simulink model "Test_MotionSM"  (R2017b)
settings: Solver=FixedStepAuto  StartTime=0.0  StopTime=inf  FixedStep=0.00001  RelTol=1e-3
model workspace (MAT data in the model file):
  AP = Simulink.Signal
  AP.DataType = 'double'
  AP.Dimensions = 1
  AP.DimensionsMode = 'Fixed'
  AP.Complexity = 'real'
  AP.SampleTime = -1
  AP.SamplingMode = 'auto'
  ZZP = Simulink.Signal
  ZZP.DataType = 'double'
  ZZP.Dimensions = 1
  ZZP.DimensionsMode = 'Fixed'
  ZZP.Complexity = 'real'
  ZZP.SampleTime = -1
  ZZP.SamplingMode = 'auto'
  ZZP.InitialValue = '0'
  ZZP_wait = Simulink.Signal
  ZZP_wait.DataType = 'double'
  ZZP_wait.Dimensions = 1
  ZZP_wait.DimensionsMode = 'Fixed'
  ZZP_wait.Complexity = 'real'
  ZZP_wait.SampleTime = -1
  ZZP_wait.SamplingMode = 'auto'
  ZZP_wait.InitialValue = '0'
settings Model: Creator=张紫薇  LastModifiedBy=张紫薇

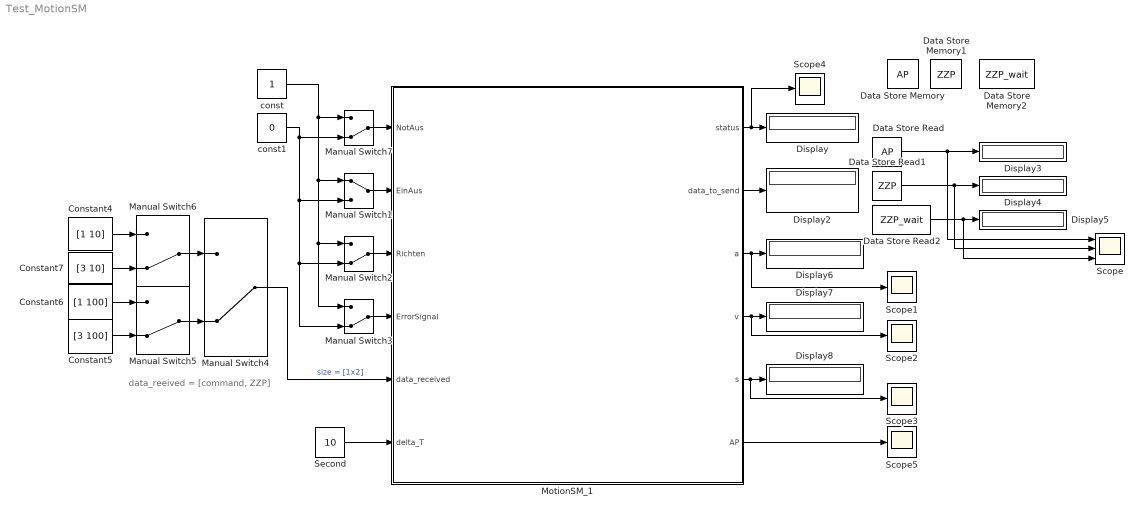
== system Test_MotionSM ==
  note: data_reeived = [command, ZZP]
  Constant4 : Constant  Value=[1 10]  OutDataTypeStr=double
  Constant5 : Constant  Value=[3 100]  OutDataTypeStr=double
  Constant6 : Constant  Value=[1 100]  OutDataTypeStr=double
  Constant7 : Constant  Value=[3 10]  OutDataTypeStr=double
  Data Store Memory : DataStoreMemory  DataStoreName=AP  ReadBeforeWriteMsg=warning  WriteAfterWriteMsg=warning  WriteAfterReadMsg=warning  ShowAdditionalParam=off  OutMin=[0]  OutMax=[100]  OutDataTypeStr=double  Dimensions=1
  Data Store Memory1 : DataStoreMemory  DataStoreName=ZZP  ReadBeforeWriteMsg=warning  WriteAfterWriteMsg=warning  WriteAfterReadMsg=warning  ShowAdditionalParam=off  OutDataTypeStr=double  Dimensions=1
  Data Store Memory2 : DataStoreMemory  DataStoreName=ZZP_wait  ReadBeforeWriteMsg=warning  WriteAfterWriteMsg=warning  WriteAfterReadMsg=warning  ShowAdditionalParam=off  OutDataTypeStr=double  Dimensions=1
  Data Store Read : DataStoreRead  DataStoreName=AP
  Data Store Read1 : DataStoreRead  DataStoreName=ZZP
  Data Store Read2 : DataStoreRead  DataStoreName=ZZP_wait
  Display{,2..8} (8 alike) : Display
      Display3 settings: Format=decimal (Stored Integer)
      Display4 settings: Format=decimal (Stored Integer)
      Display5 settings: Format=decimal (Stored Integer)
      Display8 settings: Format=decimal (Stored Integer)
  Manual Switch1 : ManualSwitch
  Manual Switch{2..7} (6 alike) : ManualSwitch  CurrentSetting=0
  MotionSM_1 : Subsystem
  Scope : Scope  NumInputPorts=3
  Scope{1..5} (5 alike) : Scope
  Second : Constant  Value=10
  const : Constant  OutDataTypeStr=boolean
  const1 : Constant  Value=0  OutDataTypeStr=boolean
  wires:
  Manual Switch4/1 -> MotionSM_1/5(data_received)  "size = [1x2]"
  const/1 -> Manual Switch3/1, Manual Switch2/1, Manual Switch1/1, Manual Switch7/1
  const1/1 -> Manual Switch3/2, Manual Switch2/2, Manual Switch1/2, Manual Switch7/2
  Manual Switch5/1 -> Manual Switch4/2
  Manual Switch7/1 -> MotionSM_1/1(NotAus)
  Manual Switch1/1 -> MotionSM_1/2(EinAus)
  Manual Switch2/1 -> MotionSM_1/3(Richten)
  Manual Switch3/1 -> MotionSM_1/4(ErrorSignal)
  MotionSM_1/1(status) -> Scope4/1, Display/1
  MotionSM_1/2(data_to_send) -> Display2/1
  Data Store Read/1 -> Scope/1, Display3/1
  Second/1 -> MotionSM_1/6(delta_T)
  Data Store Read1/1 -> Scope/2, Display4/1
  Data Store Read2/1 -> Scope/3, Display5/1
  MotionSM_1/3(a) -> Scope1/1, Display6/1
  MotionSM_1/4(v) -> Scope2/1, Display7/1
  MotionSM_1/5(s) -> Scope3/1, Display8/1
  Constant4/1 -> Manual Switch6/1
  Constant7/1 -> Manual Switch6/2
  Constant5/1 -> Manual Switch5/2
  Constant6/1 -> Manual Switch5/1
  Manual Switch6/1 -> Manual Switch4/1
  MotionSM_1/6(AP) -> Scope5/1

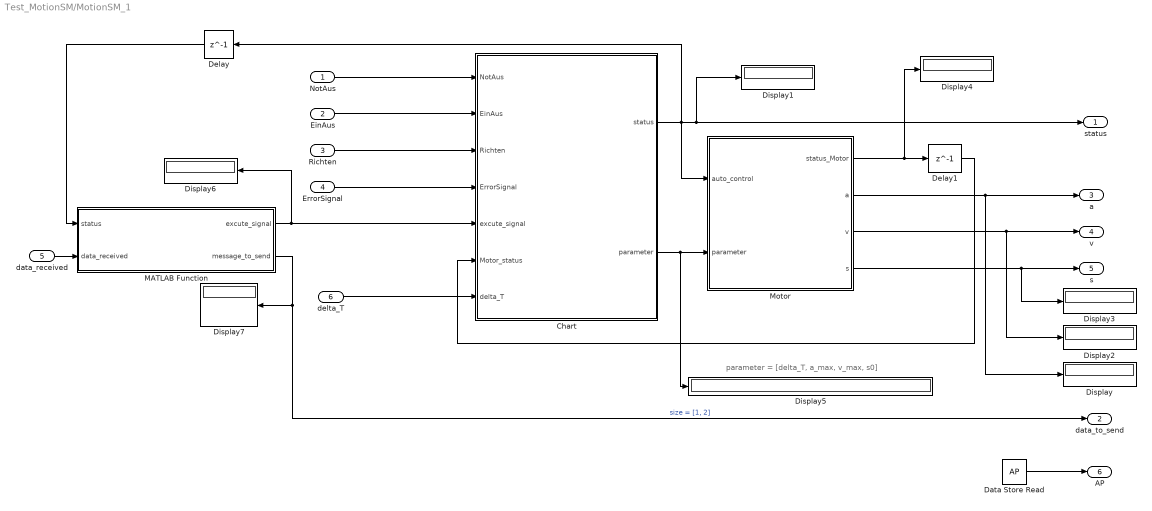
== system Test_MotionSM/MotionSM_1 ==
  note: parameter = [delta_T, a_max, v_max, s0]
  NotAus : Inport
  EinAus : Inport  Port=2
  Richten : Inport  Port=3
  ErrorSignal : Inport  Port=4
  data_received : Inport  Port=5  OutDataTypeStr=double  PortDimensions=2
  delta_T : Inport  Port=6
  Chart : Stateflow chart  TreatAsAtomicUnit=on
  Data Store Read : DataStoreRead  DataStoreName=AP
  Delay : Delay  DelayLength=1
  Delay1 : Delay  DelayLength=1
  Display{,1..7} (8 alike) : Display
  MATLAB Function : MATLAB Function  TreatAsAtomicUnit=on
  Motor : Subsystem
  status : Outport
  data_to_send : Outport  Port=2  OutDataTypeStr=double  PortDimensions=2
  a : Outport  Port=3
  v : Outport  Port=4
  s : Outport  Port=5
  AP : Outport  Port=6  OutDataTypeStr=double  PortDimensions=1
  wires:
  Chart/1(status) -> Motor/1(auto_control), Delay/1, Display1/1, status/1
  EinAus/1 -> Chart/2(EinAus)
  NotAus/1 -> Chart/1(NotAus)
  Richten/1 -> Chart/3(Richten)
  ErrorSignal/1 -> Chart/4(ErrorSignal)
  Motor/1(status_Motor) -> Display4/1, Delay1/1
  data_received/1 -> MATLAB Function/2(data_received)
  Delay1/1 -> Chart/6(Motor_status)
  MATLAB Function/1(excute_signal) -> Chart/5(excute_signal), Display6/1
  MATLAB Function/2(message_to_send) -> data_to_send/1, Display7/1  "size = [1, 2]"
  delta_T/1 -> Chart/7(delta_T)
  Motor/2(a) -> a/1, Display/1
  Motor/3(v) -> v/1, Display2/1
  Motor/4(s) -> Display3/1, s/1
  Chart/2(parameter) -> Display5/1, Motor/2(parameter)
  Delay/1 -> MATLAB Function/1(status)
  Data Store Read/1 -> AP/1

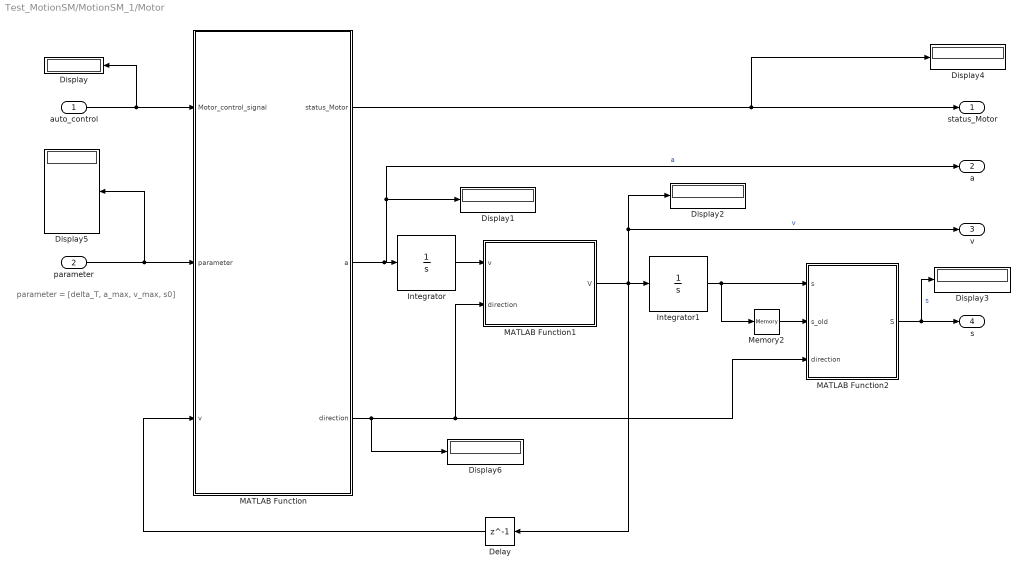
== system Test_MotionSM/MotionSM_1/Motor ==
  note: parameter = [delta_T, a_max, v_max, s0]
  auto_control : Inport
  parameter : Inport  Port=2
  Delay : Delay  DelayLength=1
  Display{,1..6} (7 alike) : Display
  Integrator : Integrator
  Integrator1 : Integrator
  MATLAB Function : MATLAB Function  TreatAsAtomicUnit=on
  MATLAB Function1 : MATLAB Function  TreatAsAtomicUnit=on
  MATLAB Function2 : MATLAB Function  TreatAsAtomicUnit=on
  Memory2 : Memory
  status_Motor : Outport
  a : Outport  Port=2
  v : Outport  Port=3
  s : Outport  Port=4
  wires:
  Integrator/1 -> MATLAB Function1/1(v)
  Integrator1/1 -> MATLAB Function2/1(s), Memory2/1
  auto_control/1 -> Display/1, MATLAB Function/1(Motor_control_signal)
  MATLAB Function/1(status_Motor) -> Display4/1, status_Motor/1
  parameter/1 -> Display5/1, MATLAB Function/2(parameter)
  MATLAB Function/2(a) -> a/1, Display1/1, Integrator/1  "a"
  MATLAB Function1/1(V) -> Display2/1, v/1, Delay/1, Integrator1/1  "v"
  MATLAB Function/3(direction) -> MATLAB Function1/2(direction), MATLAB Function2/3(direction), Display6/1
  MATLAB Function2/1(S) -> Display3/1, s/1  "s"
  Memory2/1 -> MATLAB Function2/2(s_old)
  Delay/1 -> MATLAB Function/3(v)

== matlab function Test_MotionSM/MotionSM_1/MATLAB Function ==
  data: status input double size=1; excute_signal output boolean size=1; message_to_send output double size=2; data_received input double size=2; ZZP_wait data_store_memory size=1; AP data_store_memory; ZZP data_store_memory
%data_received / message_to_send = [cmd, ZZP]
%cmd:  1...setP, 2...getP, 3...excP

function [excute_signal, message_to_send] = message_analysis(status, data_received)

global ZZP_wait
global AP
global ZZP

excute_signal = false;

cmd = data_received(1);
message_to_send = [0, 0]';

switch cmd
    case 1      %setP
        excute_signal = false;
        if ((status >= 1) && (status <= 3))
            ZZP_wait = data_received(2);
            message_to_send = [2, ZZP_wait]';
        end
        
    case 3      %excP
        excute_signal = true;
        if ((ZZP == AP) && (status == 2) && (ZZP~=ZZP_wait))
            ZZP = ZZP_wait;
        end
end
end

== matlab function Test_MotionSM/MotionSM_1/Motor/MATLAB Function ==
  settings: updateMethod=DISCRETE
  data: status_Motor output boolean size=1; Motor_control_signal input double size=1; parameter input double size=4; v input double size=1; a output double size=1; direction output double size=1; AP data_store_memory; ZZP data_store_memory
function [status_Motor, a, direction]= Motor(Motor_control_signal, parameter, v)

%delta_T = parameter(1);
a_max = abs(parameter(2));
v_max = abs(parameter(3));
s0 = parameter(4);
direction = 0;
a = 0;

s_a = 0.5 * v_max * v_max / a_max;
a_bremsen = 100000;     % 100 m/s^2

global AP
global ZZP

switch Motor_control_signal
    case {-1, 0}            %Error & Off
        if v > 0
            a = -a_bremsen;
            direction = 1;
        elseif v < 0
            a = a_bremsen;
            direction = -1;
        else
            a = 0;
            direction = 0;
        end
             
    case 1                  %Init
        if (AP > 0)
            direction = s0;
            if ((ZZP - AP) < (-s_a)) && (v > (-v_max))
                a = -a_max;
            elseif ((ZZP - AP) >= (-s_a)) && (ZZP < AP) && (v < 0)
                a = a_max;
            else
                a = 0;
            end
        else
            a = 0;
            AP = 0;
        end
        
    case 2                  %Stop
        if (v > 0)
            a = -a_max;
            direction = 1;
        elseif (v < 0)
            a = a_max;
            direction = -1;
        else
            a = 0;
            direction = 0;
        end
        
    case 3                  %run
        direction = s0;
        if (s0 > 0)   %forward
            %v_control(2) = s0;
            if ((ZZP - AP) > s_a) && (v < v_max)
                a = a_max;
            elseif ((ZZP - AP) <= s_a) && (ZZP > AP) && (v > 0)
                a = -a_max;
            else
                a = 0;
            end
        end
        if (s0 < 0)    %backward
            if ((ZZP - AP) < (-s_a)) && (v > (-v_max))
                a = -a_max;
            elseif ((ZZP - AP) >= (-s_a)) && (ZZP < AP) && (v < 0)
                a = a_max;
            else
                a = 0;
            end
        end
end
        
%status_Motor: false...Stopped, true...Running
if (a == 0) && (v == 0)
    status_Motor = false;
else
    status_Motor = true;
end

end

== stateflow chart Test_MotionSM/MotionSM_1/Chart ==
  state Off
    entry: status=0;
  state Init
    entry: status=1; parameter=Par_1(delta_T);
  state On
    state Stop
      entry: status=2;
    state Run
      entry: status=3;
    (default) -> Stop
    Stop -> Run : [excute_signal==1 && ZZP~=AP && Motor_status == 0]
        | {parameter=Par(delta_T)}
    Run -> Stop : [ZZP==AP && ~Motor_status]
  state Error
    entry: status=-1;
  (default) -> Off
  Init -> Off [order 1] : [~EinAus]
  Off -> Init [order 2] : [EinAus && ~ NotAus]{parameter=[delta_T,0,0,0]'}
  Init -> Error [order 2] : [Motor_status==-1 || NotAus || ErrorSignal]
  Off -> Error [order 1] : [EinAus && (ErrorSignal || NotAus)]
  Error -> Off [order 1] : [~EinAus]
  On -> Off [order 1] : [~EinAus]
  Error -> Init [order 2] : [Richten]{parameter=[delta_T,0,0,0]'}
  Init -> On [order 3] : [AP==0]{parameter=[delta_T,0,0,0]'}
  On -> Error [order 2] : [Motor_status==-1 || NotAus || ErrorSignal]
  data: par function_output double size=4; delta_t function_input double size=1; par function_output double size=4; delta_t function_input double size=1; NotAus input boolean size=1; EinAus input boolean size=1; Richten input boolean size=1; ErrorSignal input boolean size=1; excute_signal input boolean size=1; Motor_status input boolean size=1; status output double size=1 =0; ZZP data_store_memory; ZZP_wait data_store_memory; parameter output double size=4; AP data_store_memory size=1; delta_T input double size=1
  function par = Par_1(delta_t):
    | function par = Par_1(delta_t)
    | 
    | global ZZP
    | global ZZP_wait
    | global AP
    | 
    | % delta_T = 10 s
    | ZZP = 0;
    | ZZP_wait = 0;
    | s0 = ZZP - AP;
    | a_max = 100;        % 1 m/s^2
    | v_max = 1;
    | %v_max = 0.5 * a_max * (delta_t - sqrt(delta_t*delta_t - 4*abs(s0)/a_max));   	% mm/s
    | 
    | par = [delta_t, a_max, v_max, s0]';
    | end
  function par = Par(delta_t):
    | function par = Par(delta_t)
    | 
    | global ZZP
    | global AP
    | 
    | s0 = ZZP - AP;
    | a_max = 1000;       % 1 m/s^2
    | v_max = 0.5 * a_max * (delta_t - sqrt(delta_t*delta_t - 4*abs(s0)/a_max));  % mm/s
    | 
    | par = [delta_t, a_max, v_max, s0]';
    | end

== matlab function Test_MotionSM/MotionSM_1/Motor/MATLAB Function1 ==
  settings: updateMethod=DISCRETE
  data: V output; v input; direction input double size=1; AP data_store_memory; ZZP data_store_memory
function V = v_conrol(v, direction)

global AP
global ZZP

if direction > 0
    if ((v < 0) || (AP >= ZZP))
        V = 0;
    else
        V = v;
    end
elseif direction < 0
    if v > 0 || (AP <= ZZP)
        V = 0;
    else
        V = v;
    end
else
    V = 0;
end
end

== matlab function Test_MotionSM/MotionSM_1/Motor/MATLAB Function2 ==
  settings: updateMethod=DISCRETE
  data: s input; s_old input; S output; direction input double size=1; AP data_store_memory; ZZP data_store_memory
function S = s_control(s, s_old, direction)

global AP
global ZZP

if direction > 0
    if (AP + s - s_old) < ZZP
        S = s;
        AP = AP + s - s_old;
    else
        S = s_old;
        AP = ZZP;
    end
elseif direction < 0
    if (AP + s - s_old) > ZZP
        S = s;
        AP = AP + s - s_old;
    else
        S = s_old;
        AP = ZZP;
    end
else
    S = s_old;
end

end
